simulink model "ESP_Model"  (R2021a)
settings: Solver=VariableStepAuto  StartTime=0.0  StopTime=4  MaxStep=.001  RelTol=1e-3
values from neighbouring files (symbols this model uses):
  A_brake_piston = 0.00369    [Vehicle_Dynamics.m]
  Af = 2    [Script.m]
  alpha = 0    [Script.m]    (also in Vehicle_Dynamics.m)
  Cd = 0.3    [Script.m]
  f = 0.01    [Script.m]    (also in Vehicle_Dynamics.m = 0.015)
  g = 9.81    [Script.m]    (also in Vehicle_Dynamics.m)
  h_g = 1.3    [Script.m]
  I = 1.2    [Script.m]
  iceDistance = 20    [Script.m]
  iceTime = 1.5    [Script.m]
  L = 5    [Script.m]
  l = 2.86258    [Vehicle_Dynamics.m]
  l_f = 1.226382    [Vehicle_Dynamics.m]
  l_r = l - l_f    (= 1.636198)    [Vehicle_Dynamics.m]
  Lr = 3    [Script.m]
  m = 1908    [Script.m]    (also in Vehicle_Dynamics.m = 1818)
  mu_brakepad = 0.5    [Vehicle_Dynamics.m]
  r = 0    [Vehicle_Dynamics.m]
  r_disc = 0.1405    [Vehicle_Dynamics.m]
  rho = 1.2    [Script.m]
  Rr = 0.767/2    (= 0.3835)    [Script.m]
  v0 = 90*1000/(60*60)    (= 25)    [Script.m]
  x0 = 0    [Script.m]
undefined symbols (not defined in the file or in its folder): brake, controller, h_s, sigbuilder_block, tire, wheel_diameter
libraries: pid_lib x6, simulink x5
(part 2 of 2)

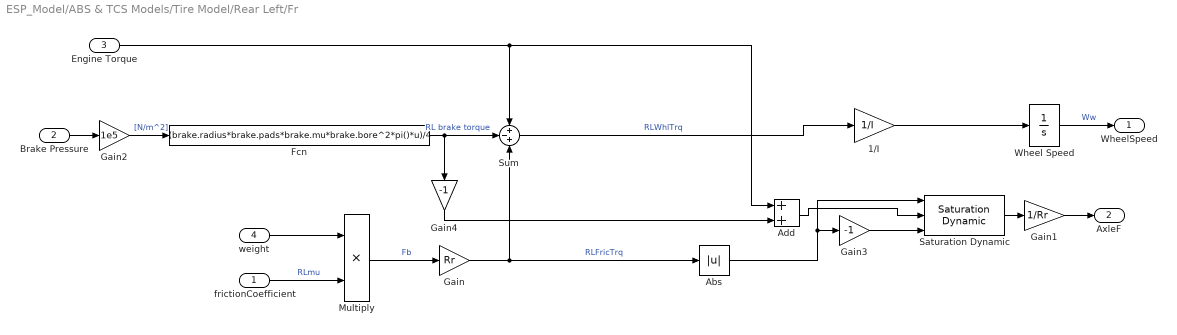
== system ESP_Model/ABS & TCS Models/Tire Model/Rear Left/Fr ==
  frictionCoefficient : Inport
  Brake Pressure : Inport  Port=2
  Engine Torque : Inport  Port=3
  weight : Inport  Port=4
  1/I : Gain  Gain=1/I  SaturateOnIntegerOverflow=on  OutDataTypeStr=Inherit: Same as input  ParamDataTypeStr=Inherit: Same as input
  Abs : Abs
  Add : Sum
  Fcn : Fcn  Expr=(brake.radius*brake.pads*brake.mu*brake.bore^2*pi()*u)/4
  Gain : Gain  Gain=Rr
  Gain1 : Gain  Gain=1/Rr
  Gain2 : Gain  Gain=1e5
  Gain3 : Gain  Gain=-1
  Gain4 : Gain  Gain=-1
  Multiply : Product
  Saturation Dynamic : simulink/Discontinuities/Saturation Dynamic  OutMin=[]  OutMax=[]  OutDataTypeStr=Inherit: Same as second input  OutDataType=fixdt(1, 16)  OutScaling=2^-10  DoSatur=off
  Sum : Sum  Inputs=+-+  InputSameDT=on  SaturateOnIntegerOverflow=on  OutDataTypeStr=Inherit: Same as first input
  Wheel Speed : Integrator  InitialCondition=v0/Rr  LimitOutput=on  UpperSaturationLimit=1000  LowerSaturationLimit=0
  WheelSpeed : Outport  VectorParamsAs1DForOutWhenUnconnected=off
  AxleF : Outport  Port=2  VectorParamsAs1DForOutWhenUnconnected=off
  wires:
  Engine Torque/1 -> Sum/1, Add/1
  1/I/1 -> Wheel Speed/1
  Brake Pressure/1 -> Gain2/1
  Fcn/1 -> Sum/2, Gain4/1  "RL brake torque"
  Wheel Speed/1 -> WheelSpeed/1  "Ww"
  weight/1 -> Multiply/1
  frictionCoefficient/1 -> Multiply/2  "RLmu"
  Multiply/1 -> Gain/1  "Fb"
  Gain/1 -> Sum/3, Abs/1  "RLFricTrq"
  Gain1/1 -> AxleF/1
  Gain2/1 -> Fcn/1  "[N/m^2]"
  Gain3/1 -> Saturation Dynamic/3
  Gain4/1 -> Add/2
  Add/1 -> Saturation Dynamic/2
  Sum/1 -> 1/I/1  "RLWhlTrq"
  Saturation Dynamic/1 -> Gain1/1
  Abs/1 -> Saturation Dynamic/1, Gain3/1

== system ESP_Model/ABS & TCS Models/Tire Model/Rear Left/Slip Model Dry ==
  VehVel (m/s) : Inport
  WheelSpeed (rad/s) : Inport  Port=2
  Bus Creator : BusCreator  Inputs=2
  Gain : Gain  Gain=1/Rr
  Relative Slip : Fcn  Expr=1.0 - u(1)/(u(2) + (u(2)==0)*eps)
  dry : Fcn  Expr=tire.dry(3)*sin(tire.dry(2)*atan((tire.dry(1)*u(1))-(tire.dry(4)*((tire.dry(1)*u(1))-atan(tire.dry(1)*u(1))))))
  mu : Outport  VectorParamsAs1DForOutWhenUnconnected=off
  wires:
  Relative Slip/1 -> dry/1  "slp"
  Bus Creator/1 -> Relative Slip/1  "yout"
  dry/1 -> mu/1
  WheelSpeed (rad/s)/1 -> Bus Creator/1
  VehVel (m/s)/1 -> Gain/1
  Gain/1 -> Bus Creator/2

== system ESP_Model/ABS & TCS Models/Tire Model/Rear Left/Slip Model Ice ==
  VehVel (m/s) : Inport
  WheelSpeed (rad/s) : Inport  Port=2
  Bus Creator : BusCreator  Inputs=2
  Gain : Gain  Gain=1/Rr
  Relative Slip : Fcn  Expr=1.0 - u(1)/(u(2) + (u(2)==0)*eps)
  ice : Fcn  Expr=tire.ice(3)*sin(tire.ice(2)*atan((tire.ice(1)*u(1))-(tire.ice(4)*((tire.ice(1)*u(1))-atan(tire.ice(1)*u(1))))))
  mu : Outport  VectorParamsAs1DForOutWhenUnconnected=off
  wires:
  WheelSpeed (rad/s)/1 -> Bus Creator/1
  ice/1 -> mu/1
  Bus Creator/1 -> Relative Slip/1  "yout"
  Relative Slip/1 -> ice/1  "RLIceslp"
  VehVel (m/s)/1 -> Gain/1
  Gain/1 -> Bus Creator/2

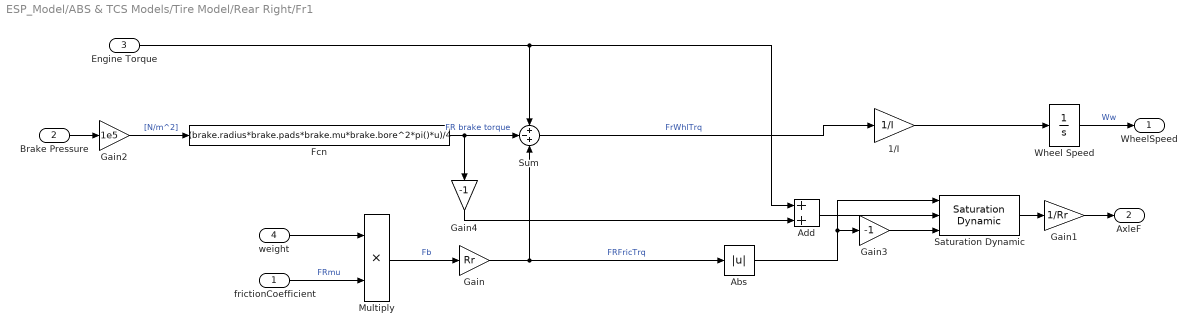
== system ESP_Model/ABS & TCS Models/Tire Model/Rear Right/Fr1 ==
  frictionCoefficient : Inport
  Brake Pressure : Inport  Port=2
  Engine Torque : Inport  Port=3
  weight : Inport  Port=4
  1/I : Gain  Gain=1/I  SaturateOnIntegerOverflow=on  OutDataTypeStr=Inherit: Same as input  ParamDataTypeStr=Inherit: Same as input
  Abs : Abs
  Add : Sum
  Fcn : Fcn  Expr=(brake.radius*brake.pads*brake.mu*brake.bore^2*pi()*u)/4
  Gain : Gain  Gain=Rr
  Gain1 : Gain  Gain=1/Rr
  Gain2 : Gain  Gain=1e5
  Gain3 : Gain  Gain=-1
  Gain4 : Gain  Gain=-1
  Multiply : Product
  Saturation Dynamic : simulink/Discontinuities/Saturation Dynamic  OutMin=[]  OutMax=[]  OutDataTypeStr=Inherit: Same as second input  OutDataType=fixdt(1, 16)  OutScaling=2^-10  DoSatur=off
  Sum : Sum  Inputs=+-+  InputSameDT=on  SaturateOnIntegerOverflow=on  OutDataTypeStr=Inherit: Same as first input
  Wheel Speed : Integrator  InitialCondition=v0/Rr  LimitOutput=on  UpperSaturationLimit=1000  LowerSaturationLimit=0
  WheelSpeed : Outport  VectorParamsAs1DForOutWhenUnconnected=off
  AxleF : Outport  Port=2  VectorParamsAs1DForOutWhenUnconnected=off
  wires:
  Engine Torque/1 -> Sum/1, Add/1
  1/I/1 -> Wheel Speed/1
  Brake Pressure/1 -> Gain2/1
  Fcn/1 -> Sum/2, Gain4/1  "FR brake torque"
  Wheel Speed/1 -> WheelSpeed/1  "Ww"
  weight/1 -> Multiply/1
  frictionCoefficient/1 -> Multiply/2  "FRmu"
  Multiply/1 -> Gain/1  "Fb"
  Gain/1 -> Sum/3, Abs/1  "FRFricTrq"
  Gain1/1 -> AxleF/1
  Gain2/1 -> Fcn/1  "[N/m^2]"
  Gain3/1 -> Saturation Dynamic/3
  Gain4/1 -> Add/2
  Sum/1 -> 1/I/1  "FrWhlTrq"
  Saturation Dynamic/1 -> Gain1/1
  Add/1 -> Saturation Dynamic/2
  Abs/1 -> Saturation Dynamic/1, Gain3/1

== system ESP_Model/ABS & TCS Models/Tire Model/Rear Right/Slip Model Dry ==
  VehVel (m/s) : Inport
  WheelSpeed (rad/s) : Inport  Port=2
  Bus Creator : BusCreator  Inputs=2
  Gain : Gain  Gain=1/Rr
  Relative Slip : Fcn  Expr=1.0 - u(1)/(u(2) + (u(2)==0)*eps)
  dry : Fcn  Expr=tire.dry(3)*sin(tire.dry(2)*atan((tire.dry(1)*u(1))-(tire.dry(4)*((tire.dry(1)*u(1))-atan(tire.dry(1)*u(1))))))
  mu : Outport  VectorParamsAs1DForOutWhenUnconnected=off
  wires:
  Relative Slip/1 -> dry/1  "slp"
  Bus Creator/1 -> Relative Slip/1  "yout"
  dry/1 -> mu/1
  WheelSpeed (rad/s)/1 -> Bus Creator/1
  VehVel (m/s)/1 -> Gain/1
  Gain/1 -> Bus Creator/2

== system ESP_Model/ABS & TCS Models/Tire Model/Rear Right/Slip Model Ice ==
  VehVel (m/s) : Inport
  WheelSpeed (rad/s) : Inport  Port=2
  Bus Creator : BusCreator  Inputs=2
  Gain : Gain  Gain=1/Rr
  Relative Slip : Fcn  Expr=1.0 - u(1)/(u(2) + (u(2)==0)*eps)
  ice : Fcn  Expr=tire.ice(3)*sin(tire.ice(2)*atan((tire.ice(1)*u(1))-(tire.ice(4)*((tire.ice(1)*u(1))-atan(tire.ice(1)*u(1))))))
  mu : Outport  VectorParamsAs1DForOutWhenUnconnected=off
  wires:
  WheelSpeed (rad/s)/1 -> Bus Creator/1
  ice/1 -> mu/1
  Bus Creator/1 -> Relative Slip/1  "yout"
  Relative Slip/1 -> ice/1  "slp"
  VehVel (m/s)/1 -> Gain/1
  Gain/1 -> Bus Creator/2
